simulink model "modelo_completo_3"  (R2023b)
settings: Solver=VariableStepAuto  StartTime=0.0  StopTime=15  FixedStep=1e-6  RelTol=1e-3
values from neighbouring files (symbols this model uses):
  P_p = 3    [constantes.m]
  tau = 0.05    [constantes.m]
  w_n_current = 6000*3    (= 18000)    [constantes.m]
  w_n_pos = 2000*3    (= 6000)    [constantes.m]
  zitta_sensor = 1    [constantes.m]
libraries: simulink x11
settings Model: Creator=Nahuel  LastModifiedBy=Nahuel

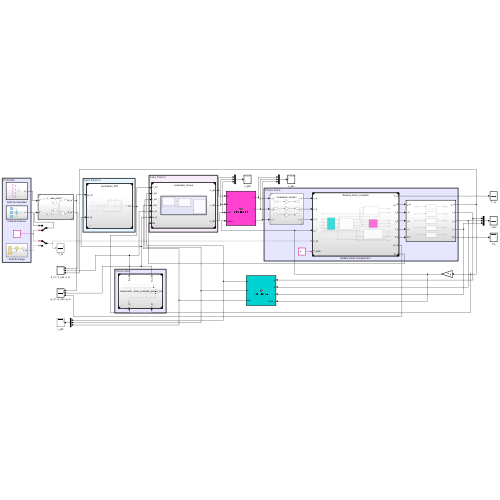
[thumbnail: Simulink's stored preview of the top-level diagram]
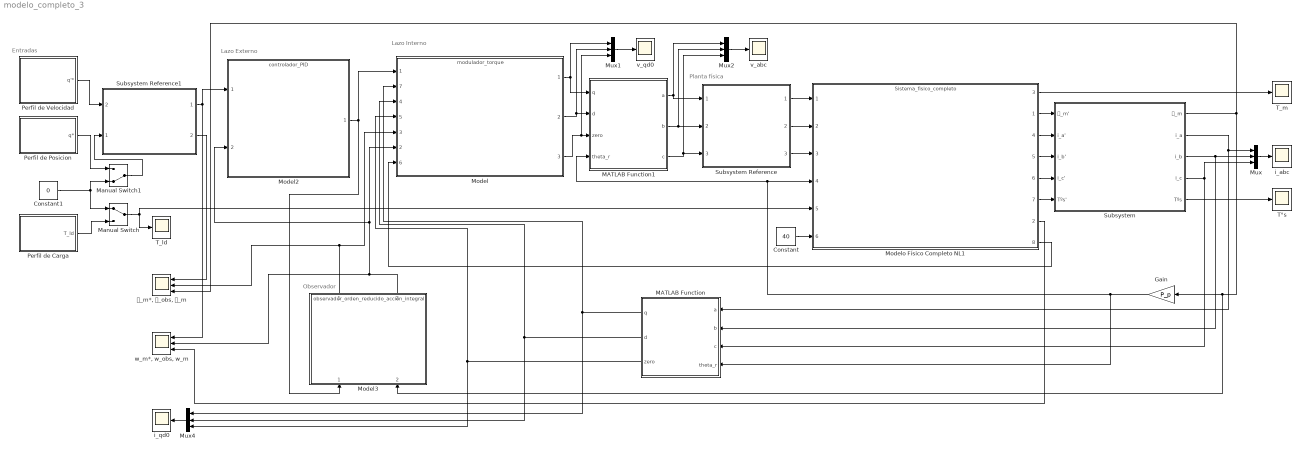
== system modelo_completo_3 ==
  note: Entradas
  note: Observador
  note: Lazo Externo
  note: Lazo Interno
  note: Planta física
  Constant : Constant  Value=40
  Constant1 : Constant  Value=0
  Gain : Gain  Gain=P_p
  MATLAB Function : MATLAB Function  TreatAsAtomicUnit=on
  MATLAB Function1 : MATLAB Function  TreatAsAtomicUnit=on
  Manual Switch : ManualSwitch
  Manual Switch1 : ManualSwitch  CurrentSetting=0
  Model : ModelReference  ModelNameDialog=modulador_torque.slx  SimulationMode=Normal  ModelReferenceVersion=1.4
      settings: PortSchema="{\"entries\":[{\"content\":{\"sides\":[{\"content\":{\"connectorIds\":[\"In1\",\"In7\",\"In4\",\"In5\",\"In3\",\"In2\",\"In6\"]},\"type\":\"ConnectorPlacement.EquallySpacedRectSide\",\"uuid\":\"1a431848-1219-464b-b81f-d5d4488f04a3\"},{\"content\":{\"connectorIds\":[\"Out1\",\"Out2\",\"Out3\"],\"side\":\"RIGHT\"},\"type\":\"ConnectorPlacement.EquallySpacedRectSide\",\"uuid\":\"e053d15c-f22a-49f8-bced-b1d540005571\"},{\"content\":{\"side\":\"TOP\"},\"type\":\"ConnectorPlacement.EquallySpacedRectSide\",\"uuid\":\"c0bb0860-826d-4b96-be85-5f71270b24f4\"}]},\"type\":\"ConnectorPlacement.EquallySpacedConnector\",\"uuid\":\"58d9e38e-69db-499f-b916-cb0043d9bf4b\"}],\"packageUris\":[\"http://schema.mathworks.com/mf0/Connector/R2020b\"],\"version\":\"1.0\"}"
  Model2 : ModelReference  ModelNameDialog=controlador_PID.slx  SimulationMode=Normal  ModelReferenceVersion=1.1
  Model3 : ModelReference  ModelNameDialog=observador_orden_reducido_accion_integral.slx  SimulationMode=Normal  ModelReferenceVersion=1.1
  Modelo Físico Completo NL1 : ModelReference  ModelNameDialog=Sistema_fisico_completo.slx  SimulationMode=Normal  ModelReferenceVersion=1.18
      settings: PortSchema="{\"entries\":[{\"content\":{\"sides\":[{\"content\":{\"connectorIds\":[\"In1\",\"In2\",\"In3\",\"In4\",\"In5\",\"In6\"]},\"type\":\"ConnectorPlacement.EquallySpacedRectSide\",\"uuid\":\"c38844a2-9b74-4da6-b9ce-d4868a84fb83\"},{\"content\":{\"connectorIds\":[\"Out3\",\"Out1\",\"Out4\",\"Out5\",\"Out6\",\"Out7\",\"Out2\",\"Out8\"],\"side\":\"RIGHT\"},\"type\":\"ConnectorPlacement.EquallySpacedRectSide\",\"uuid\":\"32cfc208-0644-4e1b-b9a9-83e6ff95cf9d\"},{\"content\":{\"side\":\"TOP\"},\"type\":\"ConnectorPlacement.EquallySpacedRectSide\",\"uuid\":\"4d8c9d59-309f-4ead-ae08-3f9c9c92e1b5\"}]},\"type\":\"ConnectorPlacement.EquallySpacedConnector\",\"uuid\":\"12663ecb-c0ca-4a2a-9423-b019766269d5\"}],\"packageUris\":[\"http://schema.mathworks.com/mf0/Connector/R2020b\"],\"version\":\"1.0\"}"
  Mux{,1..2,4} (4 alike) : Mux  Inputs=3
  Perfil de Carga : Subsystem
  Perfil de Posicion : Subsystem
  Perfil de Velocidad : Subsystem
  Subsystem : Subsystem
  Subsystem Reference : Subsystem  ReferencedSubsystem=modulador_tension
  Subsystem Reference1 : Subsystem  ReferencedSubsystem=set_point
      settings: PortSchema="{\"entries\":[{\"content\":{\"sides\":[{\"content\":{\"connectorIds\":[\"In2\",\"In1\"]},\"type\":\"ConnectorPlacement.EquallySpacedRectSide\",\"uuid\":\"88e11a35-b720-4f74-932b-4aeb2d5e00b8\"},{\"content\":{\"connectorIds\":[\"Out1\",\"Out2\"],\"side\":\"RIGHT\"},\"type\":\"ConnectorPlacement.EquallySpacedRectSide\",\"uuid\":\"e8de25d9-7d20-45a0-a221-6f807a46a39c\"},{\"content\":{\"side\":\"TOP\"},\"type\":\"ConnectorPlacement.EquallySpacedRectSide\",\"uuid\":\"c3c686d5-d3fa-4802-9f1b-650cab118ebd\"}]},\"type\":\"ConnectorPlacement.EquallySpacedConnector\",\"uuid\":\"961bc988-ee92-4957-9464-cf01ec4baf2c\"}],\"packageUris\":[\"http://schema.mathworks.com/mf0/Connector/R2020b\"],\"version\":\"1.0\"}"
  T_ld : Scope
  T_m : Scope
  T°s : Scope
  i_abc : Scope
  i_qd0 : Scope
  v_abc : Scope
  v_qd0 : Scope
  "w_m*, w_obs, w_m" : Scope  NumInputPorts=3
  "𝜃_m*, 𝜃_obs, 𝜃_m" : Scope  NumInputPorts=3
  wires:
  Subsystem Reference/1 -> Modelo Físico Completo NL1/1
  Subsystem Reference/2 -> Modelo Físico Completo NL1/2
  Subsystem Reference/3 -> Modelo Físico Completo NL1/3
  Modelo Físico Completo NL1/1 -> Subsystem/1(𝜃_m')
  Modelo Físico Completo NL1/4 -> Subsystem/2(i_a')
  Modelo Físico Completo NL1/5 -> Subsystem/3(i_b')
  Modelo Físico Completo NL1/6 -> Subsystem/4(i_c')
  Modelo Físico Completo NL1/7 -> Subsystem/5(Tºs')
  Subsystem/1(𝜃_m) -> Model3/2, Gain/1, "𝜃_m*, 𝜃_obs, 𝜃_m"/3
  Gain/1 -> Modelo Físico Completo NL1/4, MATLAB Function1/4(theta_r), MATLAB Function/4(theta_r)
  Model2/1 -> Model3/1, Model/1
  Model3/1 -> Model/3, "𝜃_m*, 𝜃_obs, 𝜃_m"/2
  Model3/2 -> Model/2, Model2/2, "w_m*, w_obs, w_m"/2
  Subsystem/2(i_a) -> MATLAB Function/1(a), Mux/1
  Subsystem/3(i_b) -> MATLAB Function/2(b), Mux/2
  Subsystem/4(i_c) -> MATLAB Function/3(c), Mux/3
  Mux/1 -> i_abc/1
  Modelo Físico Completo NL1/3 -> T_m/1
  Subsystem/5(Tºs) -> T°s/1
  MATLAB Function/1(q) -> Mux4/1, Model/7
  MATLAB Function/2(d) -> Model/4, Mux4/2
  MATLAB Function/3(zero) -> Mux4/3, Model/5
  Constant/1 -> Modelo Físico Completo NL1/6
  Model/2 -> Mux1/2, MATLAB Function1/2(d)
  Mux2/1 -> v_abc/1
  Model/3 -> MATLAB Function1/3(zero), Mux1/3
  Model/1 -> MATLAB Function1/1(q), Mux1/1
  Mux1/1 -> v_qd0/1
  MATLAB Function1/3(c) -> Subsystem Reference/3, Mux2/3
  MATLAB Function1/2(b) -> Subsystem Reference/2, Mux2/2
  MATLAB Function1/1(a) -> Subsystem Reference/1, Mux2/1
  Subsystem Reference1/2 -> "𝜃_m*, 𝜃_obs, 𝜃_m"/1
  Modelo Físico Completo NL1/8 -> Model/6
  Subsystem Reference1/1 -> Model2/1, "w_m*, w_obs, w_m"/1
  Modelo Físico Completo NL1/2 -> "w_m*, w_obs, w_m"/3
  Constant1/1 -> Manual Switch1/2, Manual Switch/1
  Perfil de Posicion/1(q*) -> Manual Switch1/1
  Perfil de Carga/1(T_ld) -> Manual Switch/2
  Manual Switch/1 -> T_ld/1, Modelo Físico Completo NL1/5
  Manual Switch1/1 -> Subsystem Reference1/1
  Perfil de Velocidad/1(q'*) -> Subsystem Reference1/2
  Mux4/1 -> i_qd0/1

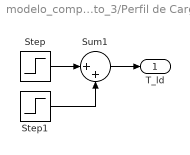
== system modelo_completo_3/Perfil de Carga ==
  Step : Step  Time=5  After=-5  SampleTime=0
  Step1 : Step  Time=10  After=10  SampleTime=0
  Sum1 : Sum  Inputs=|++
  T_ld : Outport
  wires:
  Step1/1 -> Sum1/2
  Step/1 -> Sum1/1
  Sum1/1 -> T_ld/1

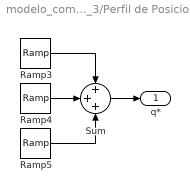
== system modelo_completo_3/Perfil de Posicion ==
  Ramp3 : simulink/Sources/Ramp  slope=2*pi/5  start=0  InitialOutput=0
  Ramp4 : simulink/Sources/Ramp  slope=-2*pi/5  start=5  InitialOutput=0
  Ramp5 : simulink/Sources/Ramp  slope=-2*pi/5  start=10  InitialOutput=0
  Sum : Sum  Inputs=+++
  q* : Outport
  wires:
  Ramp5/1 -> Sum/3
  Ramp4/1 -> Sum/2
  Ramp3/1 -> Sum/1
  Sum/1 -> q*/1

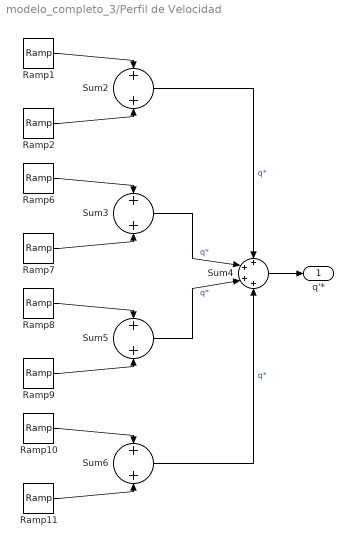
== system modelo_completo_3/Perfil de Velocidad ==
  Ramp1 : simulink/Sources/Ramp  slope=1.25/0.1  start=0  InitialOutput=0
  Ramp10 : simulink/Sources/Ramp  slope=1.25/0.1  start=14.9  InitialOutput=0
  Ramp11 : simulink/Sources/Ramp  slope=-1.25/0.1  start=15  InitialOutput=0
  Ramp2 : simulink/Sources/Ramp  slope=-1.25/0.1  start=0.1  InitialOutput=0
  Ramp6 : simulink/Sources/Ramp  slope=-1.25/0.1  start=4.9  InitialOutput=0
  Ramp7 : simulink/Sources/Ramp  slope=1.25/0.1  start=5  InitialOutput=0
  Ramp8 : simulink/Sources/Ramp  slope=-1.25/0.1  start=10  InitialOutput=0
  Ramp9 : simulink/Sources/Ramp  slope=1.25/0.1  start=10.1  InitialOutput=0
  Sum{2..3,5..6} (4 alike) : Sum
  Sum4 : Sum  Inputs=++++
  q'* : Outport
  wires:
  Ramp8/1 -> Sum5/1
  Sum6/1 -> Sum4/4  "q*"
  Ramp7/1 -> Sum3/2
  Ramp6/1 -> Sum3/1
  Ramp9/1 -> Sum5/2
  Ramp10/1 -> Sum6/1
  Ramp2/1 -> Sum2/2
  Sum3/1 -> Sum4/2  "q*"
  Sum5/1 -> Sum4/3  "q*"
  Sum2/1 -> Sum4/1  "q*"
  Ramp11/1 -> Sum6/2
  Ramp1/1 -> Sum2/1
  Sum4/1 -> q'*/1

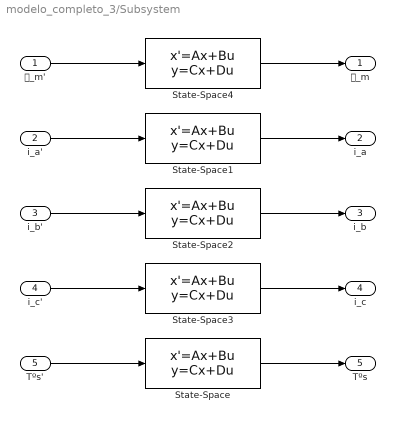
== system modelo_completo_3/Subsystem ==
  𝜃_m' : Inport
  i_a' : Inport  Port=2
  i_b' : Inport  Port=3
  i_c' : Inport  Port=4
  Tºs' : Inport  Port=5
  State-Space : StateSpace  A=[-1/tau]  B=[1/tau]  C=[1]  D=[0]  InitialCondition=40
  State-Space1 : StateSpace  A=[0 1 ; -w_n_current^2 -2*zitta_sensor*w_n_current]  B=[0; w_n_current^2]  C=[1 0]  D=[0]  InitialCondition=0
  State-Space2 : StateSpace  A=[0 1 ; -w_n_current^2 -2*zitta_sensor*w_n_current]  B=[0; w_n_current^2]  C=[1 0]  D=[0]  InitialCondition=0
  State-Space3 : StateSpace  A=[0 1 ; -w_n_current^2 -2*zitta_sensor*w_n_current]  B=[0; w_n_current^2]  C=[1 0]  D=[0]  InitialCondition=0
  State-Space4 : StateSpace  A=[0 1 ; -w_n_pos^2 -2*zitta_sensor*w_n_pos]  B=[0; w_n_pos^2]  C=[1 0]  D=[0]  InitialCondition=0
  𝜃_m : Outport
  i_a : Outport  Port=2
  i_b : Outport  Port=3
  i_c : Outport  Port=4
  Tºs : Outport  Port=5
  wires:
  i_a'/1 -> State-Space1/1
  State-Space1/1 -> i_a/1
  i_c'/1 -> State-Space3/1
  State-Space3/1 -> i_c/1
  i_b'/1 -> State-Space2/1
  State-Space2/1 -> i_b/1
  𝜃_m'/1 -> State-Space4/1
  State-Space4/1 -> 𝜃_m/1
  State-Space/1 -> Tºs/1
  Tºs'/1 -> State-Space/1

== matlab function modelo_completo_3/MATLAB Function1 ==
  data: q input; a output; d input; zero input; theta_r input; b output; c output
function [a, b, c] = park_inversa(q, d, zero, theta_r)
    % Transformación de Park Inversa
    % Entradas:
    %   d, q, z: Coordenadas en el marco rotatorio
    %   theta: Ángulo en radianes
    % Salidas:
    %   a, b, c: Valores trifásicos reconstruidos
    
    % Constantes
    alpha = 2 * pi / 3; % Desplazamiento angular entre fases
    
    % Cálculo de valores trifásicos
    a = q * cos(theta_r) + d * sin(theta_r) + zero;
    b = q * cos(theta_r - alpha) + d * sin(theta_r - alpha) + zero;
    c = q * cos(theta_r + alpha) + d * sin(theta_r + alpha) + zero;
end

== matlab function modelo_completo_3/MATLAB Function ==
  data: q output; a input; d output; b input; c input; theta_r input; zero output
function [q, d, zero] = park_directa(a, b, c, theta_r)
    % Transformación de Park Directa
    % Entradas:
    %   a, b, c: Valores trifásicos
    %   theta: Ángulo en radianes
    % Salidas:
    %   d, q, z: Coordenadas en el marco rotatorio
    
    % Constantes
    alpha = 2 * pi / 3; % Desplazamiento angular entre fases
    k = 2 / 3; % Escala para invarianza
    
    % Cálculo de coordenadas d, q, z
    q = k * (a * cos(theta_r) + b * cos(theta_r - alpha) + c * cos(theta_r + alpha));
    d = k * (a * sin(theta_r) + b * sin(theta_r - alpha) + c * sin(theta_r + alpha));
    zero = k * (a * 1/2 + b * 1/2 + c * 1/2);
end
